simulink model "simulador_01"  (R2020b)
settings: Solver=VariableStepAuto  StartTime=0.0  StopTime=T_end  RelTol=1e-3
values from neighbouring files (symbols this model uses):
  a = 1.4/255    (= 0.00549019607843)    [main_112.m]
  b = 0.03    [main_112.m]
  T_amb = 29    [main_112.m]
  t_espera = 17.5    [main_112.m]
  T_ini = 27.59    [main_112.m]
settings Model: Creator=nobel  LastModifiedBy=rober

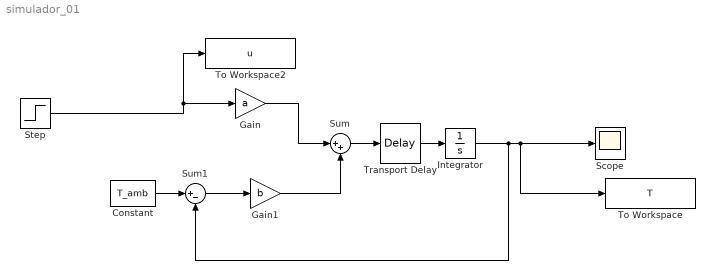
== system simulador_01 ==
  Constant : Constant  Value=T_amb
  Gain : Gain  Gain=a
  Gain1 : Gain  Gain=b
  Integrator : Integrator  InitialCondition=T_ini
  Scope : Scope
  Step : Step  Time=t_espera  Before=u  After=0  SampleTime=0
  Sum : Sum  Inputs=|++
  Sum1 : Sum  Inputs=|+-
  To Workspace : ToWorkspace  VariableName=T  SampleTime=-1
  To Workspace2 : ToWorkspace  VariableName=u  SampleTime=-1
  Transport Delay : TransportDelay  DelayTime=1.5
  wires:
  Step/1 -> To Workspace2/1, Gain/1
  Gain/1 -> Sum/1
  Constant/1 -> Sum1/1
  Sum1/1 -> Gain1/1
  Gain1/1 -> Sum/2
  Integrator/1 -> To Workspace/1, Scope/1, Sum1/2
  Sum/1 -> Transport Delay/1
  Transport Delay/1 -> Integrator/1
